simulink model "sim_car_gps_xv"  (R2022b)
settings: Solver=VariableStepAuto  StartTime=0.0  StopTime=200  RelTol=1e-3
values from neighbouring files (symbols this model uses):
  A = [1, Ts, 0, 0 ... (first row only)    [car_gps_x.m]    (also in car_gps_xv.m = [1, Ts, 0.5*Ts^2, 0, 0,  0)
  C = [1, 0, 0, 0 ... (first row only)    [car_gps_x.m]    (also in car_gps_xv.m = [1, 0, 0, 0, 0, 0)
  fgps = 10    [car_gps_x.m]    (also in car_gps_xv.m)
  Kf = Kf_t'    [car_gps_x.m]    (also in car_gps_xv.m)
  Ts = 1/fgps    (= 0.1)    [car_gps_x.m]    (also in car_gps_xv.m)
  xo_hat = [2 0 2 0]'    [car_gps_x.m]    (also in car_gps_xv.m = [2 0 0 2 0 0]')
libraries: simulink x4
settings Model: Creator=ricardoaguilera  LastModifiedBy=lucie
settings SolverCC: AlgebraicLoopSolver=TrustRegion
settings DataIOCC: ReturnWorkspaceOutputs=off
settings DebuggingCC: UnconnectedInputMsg=warning  UnconnectedOutputMsg=warning  UnconnectedLineMsg=warning  SFMachineParentedDataDiag=warning  ArithmeticOperatorsInVariantConditions=warning
settings ModelReferenceCC: EnableRefExpFcnMdlSchedulingChecks=on
settings SFSimCC: CustomCodeUndefinedFunction=UseInterfaceOnly
settings RTWCC: DLArmComputeVersion=19.05

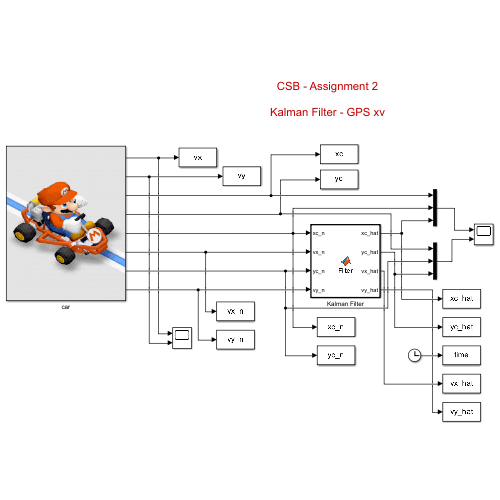
[thumbnail: Simulink's stored preview of the top-level diagram]
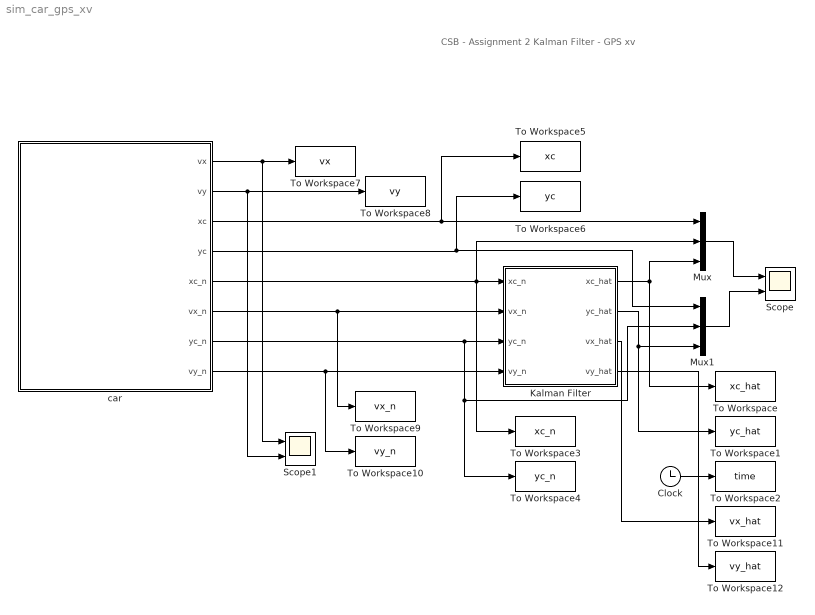
== system sim_car_gps_xv ==
  note: CSB - Assignment 2
      |
      | Kalman Filter - GPS xv
  Clock : Clock
  Kalman Filter : MATLAB Function  TreatAsAtomicUnit=on  SystemSampleTime=Ts
  Mux : Mux  Inputs=3
  Mux1 : Mux  Inputs=3
  Scope : Scope  NumInputPorts=2
  Scope1 : Scope  NumInputPorts=2
  To Workspace : ToWorkspace  VariableName=xc_hat  SampleTime=Ts
  To Workspace1 : ToWorkspace  VariableName=yc_hat  SampleTime=Ts
  To Workspace10 : ToWorkspace  VariableName=vy_n  SampleTime=Ts
  To Workspace11 : ToWorkspace  VariableName=vx_hat  SampleTime=Ts
  To Workspace12 : ToWorkspace  VariableName=vy_hat  SampleTime=Ts
  To Workspace2 : ToWorkspace  VariableName=time  SampleTime=Ts
  To Workspace3 : ToWorkspace  VariableName=xc_n  SampleTime=Ts
  To Workspace4 : ToWorkspace  VariableName=yc_n  SampleTime=Ts
  To Workspace5 : ToWorkspace  VariableName=xc  SampleTime=Ts
  To Workspace6 : ToWorkspace  VariableName=yc  SampleTime=Ts
  To Workspace7 : ToWorkspace  VariableName=vx  SampleTime=Ts
  To Workspace8 : ToWorkspace  VariableName=vy  SampleTime=Ts
  To Workspace9 : ToWorkspace  VariableName=vx_n  SampleTime=Ts
  car : Subsystem
      mask Display: image('$imagefile'); % Use "Edit Image" on toolstrip to change.
  wires:
  Kalman Filter/1(xc_hat) -> To Workspace/1, Mux/3
  Kalman Filter/2(yc_hat) -> To Workspace1/1, Mux1/3
  Mux1/1 -> Scope/2
  Clock/1 -> To Workspace2/1
  car/5(xc_n) -> To Workspace3/1, Mux/2, Kalman Filter/1(xc_n)
  car/6(vx_n) -> To Workspace9/1, Kalman Filter/2(vx_n)
  car/7(yc_n) -> Mux1/2, To Workspace4/1, Kalman Filter/3(yc_n)
  car/8(vy_n) -> To Workspace10/1, Kalman Filter/4(vy_n)
  car/3(xc) -> Mux/1, To Workspace5/1
  car/4(yc) -> Mux1/1, To Workspace6/1
  Mux/1 -> Scope/1
  car/1(vx) -> Scope1/1, To Workspace7/1
  car/2(vy) -> Scope1/2, To Workspace8/1
  Kalman Filter/3(vx_hat) -> To Workspace11/1
  Kalman Filter/4(vy_hat) -> To Workspace12/1

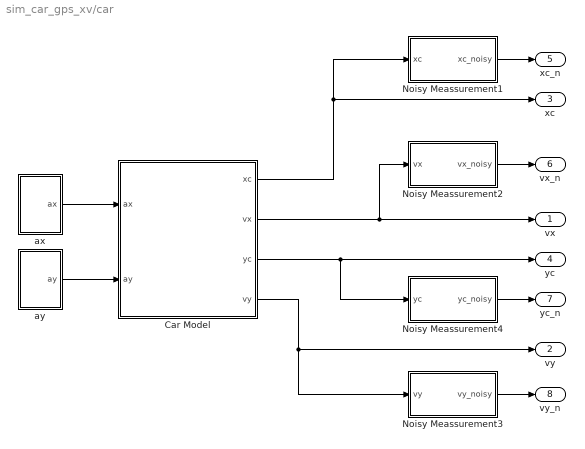
== system sim_car_gps_xv/car ==
  Car Model : MATLAB Function  TreatAsAtomicUnit=on  SystemSampleTime=0.1
  Noisy Meassurement1 : Subsystem
  Noisy Meassurement2 : Subsystem
  Noisy Meassurement3 : Subsystem
  Noisy Meassurement4 : Subsystem
  "ax " : Subsystem
  "ay " : Subsystem
  vx : Outport  VectorParamsAs1DForOutWhenUnconnected=off
  vy : Outport  Port=2  VectorParamsAs1DForOutWhenUnconnected=off
  xc : Outport  Port=3  VectorParamsAs1DForOutWhenUnconnected=off
  yc : Outport  Port=4  VectorParamsAs1DForOutWhenUnconnected=off
  xc_n : Outport  Port=5  VectorParamsAs1DForOutWhenUnconnected=off
  vx_n : Outport  Port=6  VectorParamsAs1DForOutWhenUnconnected=off
  yc_n : Outport  Port=7  VectorParamsAs1DForOutWhenUnconnected=off
  vy_n : Outport  Port=8  VectorParamsAs1DForOutWhenUnconnected=off
  wires:
  Noisy Meassurement2/1(vx_noisy) -> vx_n/1
  Noisy Meassurement3/1(vy_noisy) -> vy_n/1
  Noisy Meassurement1/1(xc_noisy) -> xc_n/1
  Noisy Meassurement4/1(yc_noisy) -> yc_n/1
  "ax "/1(ax) -> Car Model/1(ax)
  "ay "/1(ay) -> Car Model/2(ay)
  Car Model/1(xc) -> Noisy Meassurement1/1(xc), xc/1
  Car Model/2(vx) -> Noisy Meassurement2/1(vx), vx/1
  Car Model/3(yc) -> Noisy Meassurement4/1(yc), yc/1
  Car Model/4(vy) -> Noisy Meassurement3/1(vy), vy/1

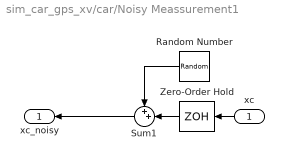
== system sim_car_gps_xv/car/Noisy Meassurement1 ==
  xc : Inport
  Random Number : RandomNumber  Variance=8  Seed=1  SampleTime=Ts
  Sum1 : Sum  Inputs=++|
  Zero-Order Hold : ZeroOrderHold  SampleTime=1/fgps
  xc_noisy : Outport  VectorParamsAs1DForOutWhenUnconnected=off
  wires:
  xc/1 -> Zero-Order Hold/1
  Zero-Order Hold/1 -> Sum1/2
  Random Number/1 -> Sum1/1
  Sum1/1 -> xc_noisy/1

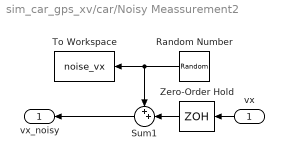
== system sim_car_gps_xv/car/Noisy Meassurement2 ==
  vx : Inport
  Random Number : RandomNumber  Variance=0.1  Seed=1  SampleTime=Ts
  Sum1 : Sum  Inputs=++|
  To Workspace : ToWorkspace  VariableName=noise_vx  SampleTime=Ts
  Zero-Order Hold : ZeroOrderHold  SampleTime=1/fgps
  vx_noisy : Outport  VectorParamsAs1DForOutWhenUnconnected=off
  wires:
  vx/1 -> Zero-Order Hold/1
  Zero-Order Hold/1 -> Sum1/2
  Random Number/1 -> Sum1/1, To Workspace/1
  Sum1/1 -> vx_noisy/1

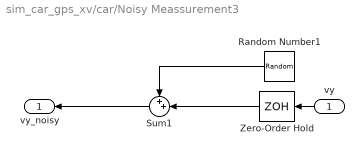
== system sim_car_gps_xv/car/Noisy Meassurement3 ==
  vy : Inport
  Random Number1 : RandomNumber  Variance=0.1  Seed=-1  SampleTime=Ts
  Sum1 : Sum  Inputs=++|
  Zero-Order Hold : ZeroOrderHold  SampleTime=1/fgps
  vy_noisy : Outport  VectorParamsAs1DForOutWhenUnconnected=off
  wires:
  vy/1 -> Zero-Order Hold/1
  Sum1/1 -> vy_noisy/1
  Random Number1/1 -> Sum1/1
  Zero-Order Hold/1 -> Sum1/2

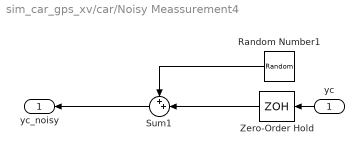
== system sim_car_gps_xv/car/Noisy Meassurement4 ==
  yc : Inport
  Random Number1 : RandomNumber  Variance=12  Seed=-1  SampleTime=Ts
  Sum1 : Sum  Inputs=++|
  Zero-Order Hold : ZeroOrderHold  SampleTime=1/fgps
  yc_noisy : Outport  VectorParamsAs1DForOutWhenUnconnected=off
  wires:
  yc/1 -> Zero-Order Hold/1
  Sum1/1 -> yc_noisy/1
  Random Number1/1 -> Sum1/1
  Zero-Order Hold/1 -> Sum1/2

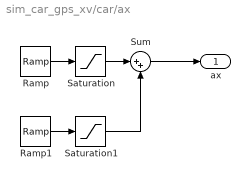
== system sim_car_gps_xv/car/ax  ==
  Ramp : simulink/Sources/Ramp  slope=30  start=10  InitialOutput=0
  Ramp1 : simulink/Sources/Ramp  slope=-100  start=20  InitialOutput=0
  Saturation : Saturate  UpperLimit=100  LowerLimit=0
  Saturation1 : Saturate  UpperLimit=1  LowerLimit=-90
  Sum : Sum  Inputs=|++
  ax : Outport  VectorParamsAs1DForOutWhenUnconnected=off
  wires:
  Ramp/1 -> Saturation/1
  Sum/1 -> ax/1
  Ramp1/1 -> Saturation1/1
  Saturation1/1 -> Sum/2
  Saturation/1 -> Sum/1

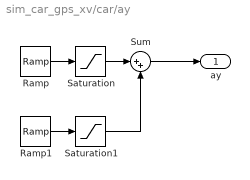
== system sim_car_gps_xv/car/ay  ==
  Ramp : simulink/Sources/Ramp  slope=500  start=35  InitialOutput=0
  Ramp1 : simulink/Sources/Ramp  slope=-50  start=40  InitialOutput=0
  Saturation : Saturate  UpperLimit=400  LowerLimit=0
  Saturation1 : Saturate  UpperLimit=0  LowerLimit=-400
  Sum : Sum  Inputs=|++
  ay : Outport  VectorParamsAs1DForOutWhenUnconnected=off
  wires:
  Ramp/1 -> Saturation/1
  Sum/1 -> ay/1
  Ramp1/1 -> Saturation1/1
  Saturation/1 -> Sum/1
  Saturation1/1 -> Sum/2

== matlab function sim_car_gps_xv/car/Car Model ==
  data: ax input; xc output; vx output; ay input; yc output; vy output
function [xc,vx,yc,vy] = fnc(ax, ay)
    [xc,vx,yc,vy] = car_vxy_model(ax,ay);
end

== matlab function sim_car_gps_xv/Kalman Filter ==
  data: xc_n input; vx_n input; yc_n input; vy_n input; A parameter; C parameter; xc_hat output; Kf parameter; yc_hat output; xo_hat parameter; vx_hat output; vy_hat output
function [xc_hat,yc_hat, vx_hat, vy_hat] = Filter(xc_n,vx_n, yc_n, vy_n, A, C, Kf,xo_hat)
% in1 to in4 are external signals
% After in4, you can add any variable from the workspace
% In "Edit Data", asign these variables as parameters.

%% Use persistent for variables that require memory
persistent x_hat_k      % Present state estimate 
    if isempty(x_hat_k) 
        x_hat_k = xo_hat;  % State estimate initialization
    end

persistent x_hat_k1         % Next-step state estimate
    if isempty(x_hat_k1)
        x_hat_k1 = xo_hat; % State estimate initialization
    end

%% Filter update 
x_hat_k=x_hat_k1;
%% Measurements

y_k=zeros(4,1);     % To create the output vector (required by Matlab)
y_k=[xc_n vx_n yc_n vy_n]';

%%  Steady-State Kalman Filter
% Implement here your Kalman Filter

y_hat_k=C*x_hat_k;
x_hat_k1 = A * x_hat_k + Kf*(y_k - y_hat_k);


xc_hat = y_hat_k(1);
yc_hat = y_hat_k(3);
vx_hat = y_hat_k(2);
vy_hat = y_hat_k(4);
